simulink model "DoubleJoints_Algorithm"  (R2018b)
settings: Solver=FixedStepDiscrete  StartTime=0.0  StopTime=Inf  FixedStep=0.001  RelTol=1e-3  EnableMultiTasking=on
undefined symbols (not defined in the file): J2, J7, Motor_Current, Motor_Position, Motor_Velocity, Send_GUIdata
libraries: c280xlib x20, simulink x9, dspsrcs4 x2, idelinklib_common x1
(part 1 of 3)
settings Model: ExtModeTrigDuration=8  Creator=jeason  LastModifiedBy=Jeason
settings SolverCC: AutoInsertRateTranBlk=on
settings OptimizationCC: DefaultUnderspecifiedDataType=single  EnhancedBackFolding=on  PassReuseOutputArgsAs=Individual arguments  MaxStackSize=512  OptimizeBlockOrder=speed  DifferentSizesBufferReuse=on  OptimizationCustomize=off
settings DebuggingCC: MultiTaskDSMMsg=none  ParameterTunabilityLossMsg=error
settings HardwareCC: ProdBitPerChar=16  ProdBitPerInt=16  ProdBitPerPointer=32  ProdBitPerSizeT=32  ProdBitPerPtrDiffT=32  ProdLargestAtomicInteger=Integer  ProdLargestAtomicFloat=None  ProdWordSize=16  ProdLongLongMode=on  ProdHWDeviceType=Texas Instruments->C2000
settings SFSimCC: MATLABDynamicMemAlloc=off
settings RTWCC: SystemTargetFile=ert.tlc  HardwareBoard=TI Delfino F2833x  TemplateMakefile=ert_default_tmf  GenerateReport=on  Toolchain=Texas Instruments Code Composer Studio (C2000)  IncludeHyperlinkInReport=on  LaunchReport=on  GenerateTraceInfo=on  GenerateTraceReport=on  GenerateTraceReportSl=on  GenerateTraceReportSf=on  GenerateTraceReportEml=on
settings CodeAppCC: ForceParamTrailComments=on  IgnoreCustomStorageClasses=off  OperatorAnnotations=on  SimulinkDataObjDesc=on  SFDataObjDesc=on  InsertBlockDesc=on
settings ERTTargetCC: CodeReplacementLibrary=TI C28x

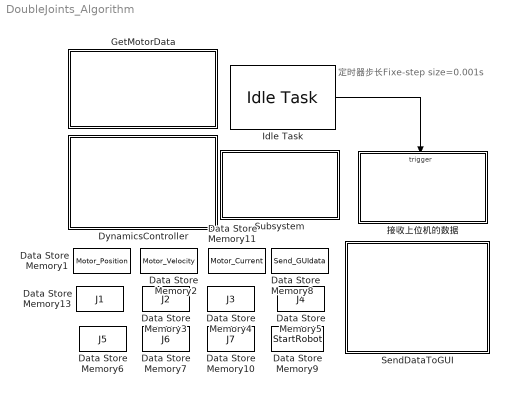
== system DoubleJoints_Algorithm ==
  note: 定时器步长Fixe-step size=0.001s
  Data Store Memory1 : DataStoreMemory  DataStoreName=Motor_Position  ReadBeforeWriteMsg=warning  WriteAfterWriteMsg=warning  WriteAfterReadMsg=warning  InitialValue=[0 0 0 0 0 0]  ShowAdditionalParam=off  OutDataTypeStr=int32
      settings: RTWStateStorageClass=ExportedGlobal
  Data Store Memory10 : DataStoreMemory  DataStoreName=J7  ReadBeforeWriteMsg=warning  WriteAfterWriteMsg=warning  WriteAfterReadMsg=warning  InitialValue=[0 0 0 0 0 0]  ShowAdditionalParam=off  OutDataTypeStr=double
      settings: RTWStateStorageClass=ExportedGlobal
  Data Store Memory11 : DataStoreMemory  DataStoreName=Motor_Current  ReadBeforeWriteMsg=warning  WriteAfterWriteMsg=warning  WriteAfterReadMsg=warning  InitialValue=[0 0 0 0 0 0]  ShowAdditionalParam=off  OutDataTypeStr=int32
      settings: RTWStateStorageClass=ExportedGlobal
  Data Store Memory13 : DataStoreMemory  DataStoreName=J1  ReadBeforeWriteMsg=warning  WriteAfterWriteMsg=warning  WriteAfterReadMsg=warning  InitialValue=[0 0 0 0 0 0]  ShowAdditionalParam=off  OutDataTypeStr=double
      settings: RTWStateStorageClass=ExportedGlobal
  Data Store Memory2 : DataStoreMemory  DataStoreName=Motor_Velocity  ReadBeforeWriteMsg=warning  WriteAfterWriteMsg=warning  WriteAfterReadMsg=warning  InitialValue=[0 0 0 0 0 0]  ShowAdditionalParam=off  OutDataTypeStr=int32
      settings: RTWStateStorageClass=ExportedGlobal
  Data Store Memory3 : DataStoreMemory  DataStoreName=J2  ReadBeforeWriteMsg=warning  WriteAfterWriteMsg=warning  WriteAfterReadMsg=warning  InitialValue=[0 0 0 0 0 0]  ShowAdditionalParam=off  OutDataTypeStr=double
      settings: RTWStateStorageClass=ExportedGlobal
  Data Store Memory4 : DataStoreMemory  DataStoreName=J3  ReadBeforeWriteMsg=warning  WriteAfterWriteMsg=warning  WriteAfterReadMsg=warning  InitialValue=[0 0 0 0 0 0]  ShowAdditionalParam=off  OutDataTypeStr=double
      settings: RTWStateStorageClass=ExportedGlobal
  Data Store Memory5 : DataStoreMemory  DataStoreName=J4  ReadBeforeWriteMsg=warning  WriteAfterWriteMsg=warning  WriteAfterReadMsg=warning  InitialValue=[0 0 0 0 0 0]  ShowAdditionalParam=off  OutDataTypeStr=double
      settings: RTWStateStorageClass=ExportedGlobal
  Data Store Memory6 : DataStoreMemory  DataStoreName=J5  ReadBeforeWriteMsg=warning  WriteAfterWriteMsg=warning  WriteAfterReadMsg=warning  InitialValue=[0 0 0 0 0 0]  ShowAdditionalParam=off  OutDataTypeStr=double
      settings: RTWStateStorageClass=ExportedGlobal
  Data Store Memory7 : DataStoreMemory  DataStoreName=J6  ReadBeforeWriteMsg=warning  WriteAfterWriteMsg=warning  WriteAfterReadMsg=warning  InitialValue=[0 0 0 0 0 0]  ShowAdditionalParam=off  OutDataTypeStr=double
      settings: RTWStateStorageClass=ExportedGlobal
  Data Store Memory8 : DataStoreMemory  DataStoreName=Send_GUIdata  ReadBeforeWriteMsg=warning  WriteAfterWriteMsg=warning  WriteAfterReadMsg=warning  InitialValue=zeros(1,18)  ShowAdditionalParam=off  OutDataTypeStr=double
      settings: RTWStateStorageClass=ExportedGlobal
  Data Store Memory9 : DataStoreMemory  DataStoreName=StartRobot  ReadBeforeWriteMsg=warning  WriteAfterWriteMsg=warning  WriteAfterReadMsg=warning  ShowAdditionalParam=off  OutDataTypeStr=uint16
      settings: RTWStateStorageClass=ExportedGlobal
  DynamicsController : Subsystem  Tag=Calculated_Data  Priority=2  TreatAsAtomicUnit=on
      settings: RTWSystemCode=Nonreusable function  RTWFcnNameOpts=Use subsystem name  RTWFileNameOpts=Use subsystem name
      mask Display:
      | color('red')
      | disp('六轴双关节\n自适应算法动力学计算')
  GetMotorData : Subsystem  Tag=Get_Data  Priority=0  TreatAsAtomicUnit=on
      settings: RTWSystemCode=Nonreusable function
  Idle Task : idelinklib_common/Idle Task  tasknumbers=[0]  taskpriorities=100016  taskpreempts=[1]  showinput=off  simPriority=0
  SendDataToGUI : Subsystem  Priority=2  TreatAsAtomicUnit=on
      settings: RTWSystemCode=Nonreusable function
  Subsystem : Subsystem
      mask Display: disp('System\nInitialization');
  接收上位机的数据 : Subsystem  TreatAsAtomicUnit=on
  wires:
  Idle Task/1 -> 接收上位机的数据/Trigger

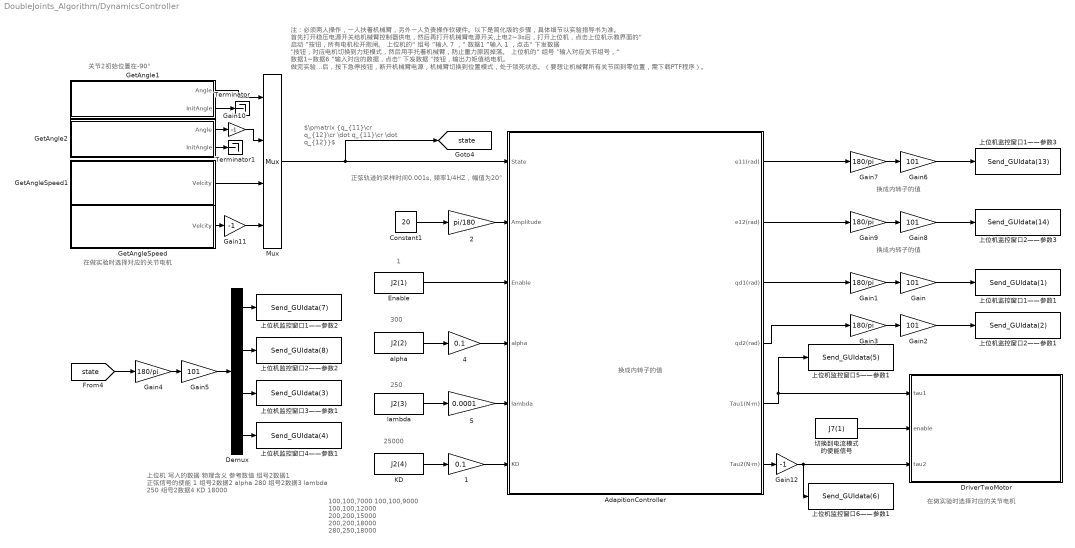
== system DoubleJoints_Algorithm/DynamicsController ==
  note: 100,100,7000
      | 100,100,9000
      | 100,100,12000
      | 200,200,15000
      | 200,200,18000
      | 280,250,18000
  note: 在做实验时选择对应的关节电机
  note: $\pmatrix {q_{11}\cr q_{12}\cr \dot q_{11}\cr \dot q_{12}}$
  note: 300
  note: 250
  note: 25000
  note: 1
  note: 在做实验时选择对应的关节电机
  note: 换成内转子的值
  note: 换成内转子的值
  note: 注：必须两人操作，一人扶着机械臂，另外一人负责操作软硬件。以下是简化版的步骤，具体细节以实验指导书为准。
      | 首先打开稳压电源开关给机械臂控制器供电，然后再打开机械臂电源开关,上电2~3s后，打开上位机，点击上位机示教界面的“ 启动 ”按钮，所有电机松开抱闸。
      | 上位机的“ 组号 ”输入 7 ，“ 数据1 ”输入 1 ，点击" 下发数据 "按钮，对应电机切换到力矩模式，然后用手托着机械臂，防止重力原因掉落。
      | 上位机的“ 组号 ”输入对应关节组号，“ 数据1~数据6 ”输入对应的数据，点击" 下发数据 "按钮，输出力矩值给电机。
      | 做完实验后，按下急停按钮，断开机械臂电源，机械臂切换到位置模式，处于锁死状态。（要想让机械臂所有关节回到零位置，需下载PTP程序）。
  note: 关节2初始位置在-90°
  note: 正弦轨迹的采样时间0.001s,
      | 频率1/4HZ，幅值为20°
  note: 上位机
      | 写入的数据
      | 物理含义
      | 参考数值
      |
      | 组号2数据1
      | 正弦信号的使能
      | 1
      |
      | 组号2数据2
      | alpha
      | 280
      |
      | 组号2数据3
      | lambda
      | 250
      |
      | 组号2数据4
      | KD
      | 18000
  note: 换成内转子的值
  1 : Gain  Gain=0.1  OutDataTypeStr=double
  2 : Gain  Gain=pi/180  OutDataTypeStr=double
  4 : Gain  Gain=0.1  OutDataTypeStr=double
  5 : Gain  Gain=0.0001  OutDataTypeStr=double
  AdapitionController : Subsystem  Priority=4  TreatAsAtomicUnit=on  RTWFcnName=AdapitionController  mask(双关节自适应算法控制器){Freq=1/4, SimpleTime=0.001}
      mask prompts: Freq "正弦信号的频率(HZ)"; SimpleTime "正弦信号的采样时间(s)"
      mask help:
      | 采样频率不能过快，否则机械臂摆动频率也会变快，至少为1/4.
      | 采样时间只能是定时器步长的整数倍，否则会报错，正弦信号的幅值最大为pi/3。
      settings: RTWSystemCode=Nonreusable function  RTWFcnNameOpts=User specified  RTWFileNameOpts=Use function name  FunctionInterfaceSpec=Allow arguments
      mask Display:
      | port_label('input', 1, 'State');
      | port_label('input', 2, '外转子正弦信号的幅值(rad)');
      | port_label('input', 3, '使能信号');
      | port_label('input', 4, 'alpha');
      | port_label('input', 5, 'lambda');
      | port_label('input', 6, 'KD');
      | 
      | port_label('output', 1, '关节2外转子跟踪误差(rad)');
      | port_label('output', 2, '关节3外转子跟踪误差(rad)');
      | port_label('output', 3, '关节2外转子理想正弦信号(rad)');
      | port_label('output', 4, '关节3外转子理想正弦信号(rad)');
      | port_label('output', 5, '关节2力矩Tau(N·m)');
      | port_label('output', 6, '关节3力矩Tau(N·m)');
  Constant1 : Constant  Value=20
  Demux : Demux
  DriverTwoMotor : Subsystem  TreatAsAtomicUnit=on  RTWFcnName=DriverTwoMotor  mask(驱动两个关节){SelectJoint1=2, SelectJoint2=3}
      mask prompts: SelectJoint1 "选择关节电机1"; SelectJoint2 "选择关节电机2"
      mask help:
      | 关节1~3为CANB,关节4~6为CANA,驱动的第一个电机的邮箱号为7，驱动的第二个电机的邮箱号为8。
      | 输入量的范围限定在-900~900。
      mask init:
      | vssBlk1_1 = [gcb, '/BottomDriver/Judgement/OneJoint/Joint1'];
      |     vssBlk1_2 = [gcb, '/BottomDriver/Judgement/OneJoint/Joint2'];
      |     vssBlk1_3 = [gcb, '/BottomDriver/Judgement/OneJoint/Joint3'];
      |     vssBlk1_4 = [gcb, '/BottomDriver/Judgement/OneJoint/Joint4'];
      |     vssBlk1_5 = [gcb, '/BottomDriver/Judgement/OneJoint/Joint5'];
      |     vssBlk1_6 = [gcb, '/BottomDriver/Judgement/OneJoint/Joint6'];
      |     vssBlk2_1 = [gcb, '/BottomDriver/Judgement/TwoJoint/Joint1'];
      |     vssBlk2_2 = [gcb, '/BottomDriver/Judgement/TwoJoint/Joint2'];
      |     vssBlk2_3 = [gcb, '/BottomDriver/Judgement/TwoJoint/Joint3'];
      |     vssBlk2_4 = [gcb, '/BottomDriver/Judgement/TwoJoint/Joint4'];
      |     vssBlk2_5 = [gcb, '/BottomDriver/Judgement/TwoJoint/Joint5'];
      |     vssBlk2_6 = [gcb, '/BottomDriver/Judgement/TwoJoint/Joint6'];
      |     choice1 = get_param(gcb,'SelectJoint1');
      |     choice2 = get_param(gcb,'SelectJoint2');
      |     if (strcmp(choice1,'1'))&&(strcmp(choice2,'1'))
      |         error('Error. Input can not be the same.');
      |     end
      |     if (strcmp(choice1,'2'))&&(strcmp(choice2,'2'))
      |         error('Error. Input can not be the same.');
      |     end
      |     if (strcmp(choice1,'3'))&&(strcmp(choice2,'3'))
      |         error('Error. Input can not be the same.');
      |     end
      |     if (strcmp(choice1,'4'))&&(strcmp(choice2,'4'))
      |         error('Error. Input can not be the same.');
      |     end
      |     if (strcmp(choice1,'5'))&&(strcmp(choice2,'5'))
      |         error('Error. Input can not be the same.');
      |     end
      |     if (strcmp(choice1,'6'))&&(strcmp(choice2,'6'))
      |         error('Error. Input can not be the same.');
      |     end
      |     clear choice1 vssBlk1_1 vssBlk1_2 vssBlk1_3 vssBlk1_4 vssBlk1_5 vssBlk1_6; 
      |     clear choice2 vssBlk2_1 vssBlk2_2 vssBlk2_3 vssBlk2_4 vssBlk2_5 vssBlk2_6;
      settings: RTWSystemCode=Nonreusable function  RTWFcnNameOpts=User specified  RTWFileNameOpts=Use function name  FunctionInterfaceSpec=Allow arguments  FunctionWithSeparateData=on
      mask TypeOptions SelectJoint1: 1 | 2 | 3 | 4 | 5 | 6
      mask Callback SelectJoint1:
      | vssBlk1_1 = [gcb, '/BottomDriver/Judgement/OneJoint/Joint1'];
      | vssBlk1_2 = [gcb, '/BottomDriver/Judgement/OneJoint/Joint2'];
      | vssBlk1_3 = [gcb, '/BottomDriver/Judgement/OneJoint/Joint3'];
      | vssBlk1_4 = [gcb, '/BottomDriver/Judgement/OneJoint/Joint4'];
      | vssBlk1_5 = [gcb, '/BottomDriver/Judgement/OneJoint/Joint5'];
      | vssBlk1_6 = [gcb, '/BottomDriver/Judgement/OneJoint/Joint6'];
      | choice1 = get_param(gcb,'SelectJoint1');
      | if strcmp(choice1,'1')
      |     set_param(vssBlk1_1, 'Commented','off');
      |     set_param(vssBlk1_2,'Commented','on');
      |     set_param(vssBlk1_3,'Commented','on');
      |     set_param(vssBlk1_4,'Commented','on');
      |     set_param(vssBlk1_5,'Commented','on');
      |     set_param(vssBlk1_6,'Commented','on');
      | elseif strcmp(choice1,'2')
      |     set_param(vssBlk1_2, 'Commented','off');
      |     set_param(vssBlk1_1,'Commented','on');
      |     set_param(vssBlk1_3,'Commented','on');
      |     set_param(vssBlk1_4,'Commented','on');
      |     set_param(vssBlk1_5,'Commented','on');
      |     set_param(vssBlk1_6,'Commented','on');
      | elseif strcmp(choice1,'3')
      |     set_param(vssBlk1_3, 'Commented','off');
      |     set_param(vssBlk1_1,'Commented','on');
      |     set_param(vssBlk1_2,'Commented','on');
      |     set_param(vssBlk1_4,'Commented','on');
      |     set_param(vssBlk1_5,'Commented','on');
      |     set_param(vssBlk1_6,'Commented','on');
      | elseif strcmp(choice1,'4')
      |     set_param(vssBlk1_4, 'Commented','off');
      |     set_param(vssBlk1_1,'Commented','on');
      |     set_param(vssBlk1_2,'Commented','on');
      |     set_param(vssBlk1_3,'Commented','on');
      |     set_param(vssBlk1_5,'Commented','on');
      |     set_param(vssBlk1_6,'Commented','on');
      | elseif strcmp(choice1,'5')
      |     set_param(vssBlk1_5, 'Commented','off');
      |     set_param(vssBlk1_1,'Commented','on');
      |     set_param(vssBlk1_2,'Commented','on');
      |     set_param(vssBlk1_3,'Commented','on');
      |     set_param(vssBlk1_4,'Commented','on');
      |     set_param(vssBlk1_6,'Commented','on');
      | elseif strcmp(choice1,'6')
      |     set_param(vssBlk1_6, 'Commented','off');
      |     set_param(vssBlk1_1,'Commented','on');
      |     set_param(vssBlk1_2,'Commented','on');
      |     set_param(vssBlk1_3,'Commented','on');
      |     set_param(vssBlk1_4,'Commented','on');
      |     set_param(vssBlk1_5,'Commented','on');
      | end
      | clear choice1 vssBlk1_1 vssBlk1_2 vssBlk1_3 vssBlk1_4 vssBlk1_5 vssBlk1_6;
      mask TypeOptions SelectJoint2: 1 | 2 | 3 | 4 | 5 | 6
      mask Callback SelectJoint2:
      | vssBlk2_1 = [gcb, '/BottomDriver/Judgement/TwoJoint/Joint1'];
      | vssBlk2_2 = [gcb, '/BottomDriver/Judgement/TwoJoint/Joint2'];
      | vssBlk2_3 = [gcb, '/BottomDriver/Judgement/TwoJoint/Joint3'];
      | vssBlk2_4 = [gcb, '/BottomDriver/Judgement/TwoJoint/Joint4'];
      | vssBlk2_5 = [gcb, '/BottomDriver/Judgement/TwoJoint/Joint5'];
      | vssBlk2_6 = [gcb, '/BottomDriver/Judgement/TwoJoint/Joint6'];
      | choice2 = get_param(gcb,'SelectJoint2');
      |  if strcmp(choice2,'1')
      |     set_param(vssBlk2_1, 'Commented','off');
      |     set_param(vssBlk2_2,'Commented','on');
      |     set_param(vssBlk2_3,'Commented','on');
      |     set_param(vssBlk2_4,'Commented','on');
      |     set_param(vssBlk2_5,'Commented','on');
      |     set_param(vssBlk2_6,'Commented','on');
      | elseif strcmp(choice2,'2')
      |     set_param(vssBlk2_2, 'Commented','off');
      |     set_param(vssBlk2_1,'Commented','on');
      |     set_param(vssBlk2_3,'Commented','on');
      |     set_param(vssBlk2_4,'Commented','on');
      |     set_param(vssBlk2_5,'Commented','on');
      |     set_param(vssBlk2_6,'Commented','on');
      | elseif strcmp(choice2,'3')
      |     set_param(vssBlk2_3, 'Commented','off');
      |     set_param(vssBlk2_1,'Commented','on');
      |     set_param(vssBlk2_2,'Commented','on');
      |     set_param(vssBlk2_4,'Commented','on');
      |     set_param(vssBlk2_5,'Commented','on');
      |     set_param(vssBlk2_6,'Commented','on');
      | elseif strcmp(choice2,'4')
      |     set_param(vssBlk2_4, 'Commented','off');
      |     set_param(vssBlk2_1,'Commented','on');
      |     set_param(vssBlk2_2,'Commented','on');
      |     set_param(vssBlk2_3,'Commented','on');
      |     set_param(vssBlk2_5,'Commented','on');
      |     set_param(vssBlk2_6,'Commented','on');
      | elseif strcmp(choice2,'5')
      |     set_param(vssBlk2_5, 'Commented','off');
      |     set_param(vssBlk2_1,'Commented','on');
      |     set_param(vssBlk2_2,'Commented','on');
      |     set_param(vssBlk2_3,'Commented','on');
      |     set_param(vssBlk2_4,'Commented','on');
      |     set_param(vssBlk2_6,'Commented','on');
      | elseif strcmp(choice2,'6')
      |     set_param(vssBlk2_6, 'Commented','off');
      |     set_param(vssBlk2_1,'Commented','on');
      |     set_param(vssBlk2_2,'Commented','on');
      |     set_param(vssBlk2_3,'Commented','on');
      |     set_param(vssBlk2_4,'Commented','on');
      |     set_param(vssBlk2_5,'Commented','on');
      | end
      | clear choice2 vssBlk2_1 vssBlk2_2 vssBlk2_3 vssBlk2_4 vssBlk2_5 vssBlk2_6;
      mask Display:
      | str1='双关节算法';str2='驱动关节'; str3='和';str4='电机';
      | choice1 = get_param(gcb,'SelectJoint1');
      | choice2 = get_param(gcb,'SelectJoint2');
      | str=[str1,'\n',str2,choice1,str3,choice2,str4];
      | disp(str);
      | port_label('input', 1, 'Tau1');
      | port_label('input', 2, 'Enable');
      | port_label('input', 3, 'Tau2');
  Enable : DataStoreRead  DataStoreName=J2  DataStoreElements=J2(1)
  Gain{,2,5..6,8} (5 alike) : Gain  Gain=101
  Gain{1,3..4,7,9} (5 alike) : Gain  Gain=180/pi
  Gain10 : Gain  Gain=-1
  Gain11 : Gain  Gain=-1
  Gain12 : Gain  Gain=-1
  GetAngle1 : Subsystem  TreatAsAtomicUnit=on  mask(获取电机外转子角度(rad)){JJoint=2, InitAngle=-90}
      mask prompts: JJoint "选择关节电机"; InitAngle "给定初始角度(deg)"
      mask help:
      | 给定初始角度：假设在数学建模时，设定连杆在水平位置为0°，而机械臂每个关节在出厂时都设定在竖直位置为0°，那么这里就需要给定一个偏置值90°/-90°，默认设为0。
      | 注：关节3因为结构原因实际获取到的角度的正负和标签贴的方向相反。
      | Angle(rad)=电机外转子的实际角度值-给定的初始角度值
      | InitAngle(rad)=给定的初始角度值
      mask TypeOptions JJoint: 1 | 2 | 3 | 4 | 5 | 6
      mask Display:
      | choice1 = get_param(gcb,'JJoint');
      | color('black');
      | switch choice1
      |     case '1'
      |         disp('获取关节1电机\n外转子角度(rad)');
      |     case '2'
      |         disp('获取关节2电机\n外转子角度(rad)');
      |     case '3'
      |         disp('获取关节3电机\n外转子角度(rad)');
      |     case '4'
      |         disp('获取关节4电机\n外转子角度(rad)');
      |     case '5'
      |         disp('获取关节5电机\n外转子角度(rad)');
      |     case '6'
      |         disp('获取关节6电机\n外转子角度(rad)');
      | end
      | color('black');
      | port_label('output', 1, 'Angle');
      | port_label('output', 2, 'InitAngle');
      | clear choice1;
  GetAngle2 : Subsystem  TreatAsAtomicUnit=on  mask(获取电机外转子角度(rad)){JJoint=3, InitAngle=0}
      mask prompts: JJoint "选择关节电机"; InitAngle "给定初始角度(deg)"
      mask help:
      | 给定初始角度：假设在数学建模时，设定连杆在水平位置为0°，而机械臂每个关节在出厂时都设定在竖直位置为0°，那么这里就需要给定一个偏置值90°/-90°，默认设为0。
      | 注：关节3因为结构原因实际获取到的角度的正负和标签贴的方向相反。
      | Angle(rad)=电机外转子的实际角度值-给定的初始角度值
      | InitAngle(rad)=给定的初始角度值
      mask TypeOptions JJoint: 1 | 2 | 3 | 4 | 5 | 6
      mask Display:
      | choice1 = get_param(gcb,'JJoint');
      | color('black');
      | switch choice1
      |     case '1'
      |         disp('获取关节1电机\n外转子角度(rad)');
      |     case '2'
      |         disp('获取关节2电机\n外转子角度(rad)');
      |     case '3'
      |         disp('获取关节3电机\n外转子角度(rad)');
      |     case '4'
      |         disp('获取关节4电机\n外转子角度(rad)');
      |     case '5'
      |         disp('获取关节5电机\n外转子角度(rad)');
      |     case '6'
      |         disp('获取关节6电机\n外转子角度(rad)');
      | end
      | color('black');
      | port_label('output', 1, 'Angle');
      | port_label('output', 2, 'InitAngle');
      | clear choice1;
  GetAngleSpeed : Subsystem  TreatAsAtomicUnit=on  mask{JJoint=3}
      mask prompts: JJoint "选择关节电机"
      mask help: 读取电机角速度(rad/s)
      mask TypeOptions JJoint: 1 | 2 | 3 | 4 | 5 | 6
      mask Display:
      | choice1 = get_param(gcb,'JJoint');
      | color('black');
      | switch choice1
      |     case '1'
      |         disp('获取关节1电机\n外转子角速度(rad/s)');
      |     case '2'
      |         disp('获取关节2电机\n外转子角速度(rad/s)');
      |     case '3'
      |         disp('获取关节3电机\n外转子角速度(rad/s)');
      |     case '4'
      |         disp('获取关节4电机\n外转子角速度(rad/s)');
      |     case '5'
      |         disp('获取关节5电机\n外转子角速度(rad/s)');
      |     case '6'
      |         disp('获取关节6电机\n外转子角速度(rad/s)');
      | end
      | color('black');
      | port_label('output', 1, 'Velocity');
      | clear choice1;
  GetAngleSpeed1 : Subsystem  TreatAsAtomicUnit=on  mask{JJoint=2}
      mask prompts: JJoint "选择关节电机"
      mask help: 读取电机角速度(rad/s)
      mask TypeOptions JJoint: 1 | 2 | 3 | 4 | 5 | 6
      mask Display:
      | choice1 = get_param(gcb,'JJoint');
      | color('black');
      | switch choice1
      |     case '1'
      |         disp('获取关节1电机\n外转子角速度(rad/s)');
      |     case '2'
      |         disp('获取关节2电机\n外转子角速度(rad/s)');
      |     case '3'
      |         disp('获取关节3电机\n外转子角速度(rad/s)');
      |     case '4'
      |         disp('获取关节4电机\n外转子角速度(rad/s)');
      |     case '5'
      |         disp('获取关节5电机\n外转子角速度(rad/s)');
      |     case '6'
      |         disp('获取关节6电机\n外转子角速度(rad/s)');
      | end
      | color('black');
      | port_label('output', 1, 'Velocity');
      | clear choice1;
  KD : DataStoreRead  DataStoreName=J2  DataStoreElements=J2(4)
  Mux : Mux
  Terminator : Terminator
  Terminator1 : Terminator
  alpha : DataStoreRead  DataStoreName=J2  DataStoreElements=J2(2)
  lambda : DataStoreRead  DataStoreName=J2  DataStoreElements=J2(3)
  上位机监控窗口1——参数1 : DataStoreWrite  DataStoreName=Send_GUIdata  DataStoreElements=Send_GUIdata(1)
  上位机监控窗口1——参数2 : DataStoreWrite  DataStoreName=Send_GUIdata  DataStoreElements=Send_GUIdata(7)
  上位机监控窗口1——参数3 : DataStoreWrite  DataStoreName=Send_GUIdata  DataStoreElements=Send_GUIdata(13)
  上位机监控窗口2——参数1 : DataStoreWrite  DataStoreName=Send_GUIdata  DataStoreElements=Send_GUIdata(2)
  上位机监控窗口2——参数2 : DataStoreWrite  DataStoreName=Send_GUIdata  DataStoreElements=Send_GUIdata(8)
  上位机监控窗口2——参数3 : DataStoreWrite  DataStoreName=Send_GUIdata  DataStoreElements=Send_GUIdata(14)
  上位机监控窗口3——参数1 : DataStoreWrite  DataStoreName=Send_GUIdata  DataStoreElements=Send_GUIdata(3)
  上位机监控窗口4——参数1 : DataStoreWrite  DataStoreName=Send_GUIdata  DataStoreElements=Send_GUIdata(4)
  上位机监控窗口5——参数1 : DataStoreWrite  DataStoreName=Send_GUIdata  DataStoreElements=Send_GUIdata(5)
  上位机监控窗口6——参数1 : DataStoreWrite  DataStoreName=Send_GUIdata  DataStoreElements=Send_GUIdata(6)
  切换到电流模式 的使能信号 : DataStoreRead  DataStoreName=J7  DataStoreElements=J7(1)
  tag scope: state=global
  wires:
  KD/1 -> 1/1
  Constant1/1 -> 2/1
  GetAngle1/1(Angle) -> Mux/1
  GetAngleSpeed1/1(Velcity) -> Mux/3
  GetAngleSpeed/1(Velcity) -> Gain11/1
  切换到电流模式 的使能信号/1 -> DriverTwoMotor/2(enable)
  Gain1/1 -> Gain/1
  Gain/1 -> 上位机监控窗口1——参数1/1
  Gain3/1 -> Gain2/1
  Gain2/1 -> 上位机监控窗口2——参数1/1
  Demux/1 -> 上位机监控窗口1——参数2/1
  Demux/2 -> 上位机监控窗口2——参数2/1
  [state] -> Gain4/1
  Gain4/1 -> Gain5/1
  Gain5/1 -> Demux/1
  Gain9/1 -> Gain8/1
  Gain7/1 -> Gain6/1
  Gain6/1 -> 上位机监控窗口1——参数3/1
  Gain8/1 -> 上位机监控窗口2——参数3/1
  Demux/4 -> 上位机监控窗口4——参数1/1
  Demux/3 -> 上位机监控窗口3——参数1/1
  AdapitionController/6(Tau2(N·m)) -> Gain12/1
  AdapitionController/5(Tau1(N·m)) -> DriverTwoMotor/1(tau1), 上位机监控窗口5——参数1/1
  Mux/1 -> AdapitionController/1(State), [state]
  2/1 -> AdapitionController/2(Amplitude)
  4/1 -> AdapitionController/4(alpha)
  5/1 -> AdapitionController/5(lambda)
  1/1 -> AdapitionController/6(KD)
  AdapitionController/1(e11(rad)) -> Gain7/1
  AdapitionController/2(e12(rad)) -> Gain9/1
  AdapitionController/3(qd1(rad)) -> Gain1/1
  AdapitionController/4(qd2(rad)) -> Gain3/1
  Gain10/1 -> Mux/2
  Gain11/1 -> Mux/4
  Gain12/1 -> DriverTwoMotor/3(tau2), 上位机监控窗口6——参数1/1
  lambda/1 -> 5/1
  alpha/1 -> 4/1
  Enable/1 -> AdapitionController/3(Enable)
  GetAngle2/1(Angle) -> Gain10/1
  GetAngle1/2(InitAngle) -> Terminator/1
  GetAngle2/2(InitAngle) -> Terminator1/1

== system DoubleJoints_Algorithm/GetMotorData ==
  note: 获取关节电流、 角速度、 角度信息
  CANA_284_24 : Subsystem  Priority=4  TreatAsAtomicUnit=on
      settings: RTWSystemCode=Nonreusable function
      mask Display:
      | color('WHITE')
      | disp('JOINT4\n数据读取')
  CANA_285_25 : Subsystem  Priority=5  TreatAsAtomicUnit=on
      settings: RTWSystemCode=Nonreusable function
      mask Display:
      | color('WHITE')
      | disp('JOINT5\n数据读取')
  CANA_286_26 : Subsystem  Priority=6  TreatAsAtomicUnit=on
      settings: RTWSystemCode=Nonreusable function
      mask Display:
      | color('WHITE')
      | disp('JOINT6\n数据读取')
  CANB_281_21 : Subsystem  Priority=1  TreatAsAtomicUnit=on
      settings: RTWSystemCode=Nonreusable function
      mask Display:
      | color('WHITE')
      | disp('JOINT1\n数据读取')
  CANB_282_22 : Subsystem  Priority=2  TreatAsAtomicUnit=on
      settings: RTWSystemCode=Nonreusable function
      mask Display:
      | color('white')
      | disp('JOINT2\n数据读取')
  CANB_283_23 : Subsystem  Priority=3  TreatAsAtomicUnit=on
      settings: RTWSystemCode=Nonreusable function
      mask Display:
      | color('white')
      | disp('JOINT3\n数据读取')

== system DoubleJoints_Algorithm/SendDataToGUI ==
  note: Upper limit=9
  note: 发送数据给上位机
  note: 定时器步长Fixe-step size=0.001s,
      | 每10ms发送一次数据给上位机
  " " : Subsystem
  Constant : Constant  Value=true  OutDataTypeStr=boolean
  Constant1 : Constant  Value=false  OutDataTypeStr=boolean
  Switch : Switch  Criteria=u2 > Threshold
  广播周期 : simulink/Sources/Counter Limited  uplimit=9  tsamp=-1
  wires:
  Switch/1 -> " "/Enable
  广播周期/1 -> Switch/2
  Constant1/1 -> Switch/1
  Constant/1 -> Switch/3

== system DoubleJoints_Algorithm/Subsystem ==
  Model Header : Subsystem  mask(Model Header){ShowInLibBrowser=0}
      mask prompts: ShowInLibBrowser "Simulink:masks:CustCodeMaskParam1_MP"
      settings: CopyFcn=cccopyfcn(gcb)  OpenFcn=ccopenfcn('Model Header')
      mask Help: eval('feval(''rtwprivate'',''rtwhelpview'',''rtw_model_header_block'')');
      mask Display: disp('Model\nHeader');
  Model Source : Subsystem  mask(Model Source){ShowInLibBrowser=0}
      mask prompts: ShowInLibBrowser "Simulink:masks:CustCodeMaskParam1_MP"
      settings: CopyFcn=cccopyfcn(gcb)  OpenFcn=ccopenfcn('Model Source')
      mask Help: eval('feval(''rtwprivate'',''rtwhelpview'',''rtw_model_source_block'')');
      mask Display: disp('Model\nSource');
  System Initialize : Subsystem  mask(System Initialize){ShowInLibBrowser=0}
      mask prompts: ShowInLibBrowser "Simulink:masks:CustCodeMaskParam1_MP"
      settings: CopyFcn=cccopyfcn(gcb)  OpenFcn=ccopenfcn('System Initialize Function')
      mask Help: eval('feval(''rtwprivate'',''rtwhelpview'',''rtw_sys_initialize_block'')');
      mask Display: disp('System\nInitialize');

== system DoubleJoints_Algorithm/接收上位机的数据 ==
  note: 接收上位机数据
  function : TriggerPort  TriggerType=function-call  VariantControl=Variant
  0x0080 : simulink/Logic and Bit Operations/Compare To Constant  relop===  const=hex2dec('0080')  OutDataTypeStr=boolean
  0x88 : simulink/Logic and Bit Operations/Compare To Constant  relop===  const=hex2dec('0088')  OutDataTypeStr=boolean
  Compare To Constant1 : simulink/Logic and Bit Operations/Compare To Constant  relop===  const=hex2dec('0001')  OutDataTypeStr=boolean
  Compare To Constant2 : simulink/Logic and Bit Operations/Compare To Constant  relop===  const=hex2dec('0001')  OutDataTypeStr=boolean
  Data Store Read : DataStoreRead  DataStoreName=PTX
  Data Store Write2 : DataStoreWrite  DataStoreName=StartRobot
  Data Type Conversion : DataTypeConversion  OutDataTypeStr=int16
  Data Type Conversion3 : DataTypeConversion  OutDataTypeStr=double
  Data Type Conversion4 : DataTypeConversion  OutDataTypeStr=uint16
  Demux1 : Demux  Outputs=9
  Logical Operator : Logic  Inputs=4  AllPortsSameDT=off  OutDataTypeStr=boolean
  Mux1 : Mux  Inputs=6
  Subsystem : Subsystem
  Terminator3 : Terminator
  消息使能 : DataStoreMemory  DataStoreName=PTX  ReadBeforeWriteMsg=warning  WriteAfterWriteMsg=warning  WriteAfterReadMsg=warning  InitialValue=true  ShowAdditionalParam=off  OutDataTypeStr=boolean
  获取用户命令 : Subsystem  Priority=1  TreatAsAtomicUnit=on
      settings: RTWSystemCode=Nonreusable function
  wires:
  Compare To Constant2/1 -> Logical Operator/4
  Compare To Constant1/1 -> Logical Operator/3
  Data Store Read/1 -> Logical Operator/2
  Logical Operator/1 -> Data Type Conversion4/1
  0x0080/1 -> Logical Operator/1
  Demux1/4 -> Mux1/2, Compare To Constant2/1
  Demux1/3 -> Mux1/1, Compare To Constant1/1
  Demux1/1 -> 0x0080/1, 0x88/1
  获取用户命令/1(消息) -> Demux1/1
  Demux1/5 -> Mux1/3
  Demux1/6 -> Mux1/4
  Demux1/9 -> Terminator3/1
  Demux1/7 -> Mux1/5
  Demux1/8 -> Mux1/6
  Mux1/1 -> Data Type Conversion/1
  Data Type Conversion/1 -> Data Type Conversion3/1
  Data Type Conversion4/1 -> Data Store Write2/1
  Demux1/2 -> Subsystem/1(组号)
  Data Type Conversion3/1 -> Subsystem/2(数据)
  0x88/1 -> Subsystem/Enable

== system DoubleJoints_Algorithm/DynamicsController/AdapitionController ==
  State : Inport
  Amplitude : Inport  Port=2
  Enable : Inport  Port=3
  alpha : Inport  Port=4
  lambda : Inport  Port=5
  KD : Inport  Port=6
  Controller : Subsystem  Priority=1  TreatAsAtomicUnit=on
      settings: RTWSystemCode=Nonreusable function  FunctionInterfaceSpec=Allow arguments
  "Error " : Subsystem  Priority=0  TreatAsAtomicUnit=on
      settings: RTWSystemCode=Nonreusable function  FunctionInterfaceSpec=Allow arguments
  Saturation : Saturate  UpperLimit=pi/3  LowerLimit=0
  e11(rad) : Outport
  e12(rad) : Outport  Port=2
  qd1(rad) : Outport  Port=3
  qd2(rad) : Outport  Port=4
  Tau1(N·m) : Outport  Port=5
  Tau2(N·m) : Outport  Port=6
  wires:
  "Error "/9(s1) -> Controller/6(s1)
  "Error "/7(ddqr1) -> Controller/4(ddqr_1)
  State/1 -> Controller/1(q), "Error "/1(state)
  Amplitude/1 -> Saturation/1
  "Error "/4(qd2) -> qd2(rad)/1
  "Error "/10(s2) -> Controller/7(s2)
  "Error "/8(ddqr2) -> Controller/5(ddqr_2)
  "Error "/5(dqr1) -> Controller/2(dqr_1)
  KD/1 -> Controller/9(KD)
  "Error "/6(dqr2) -> Controller/3(dqr_2)
  "Error "/3(qd1) -> qd1(rad)/1
  alpha/1 -> "Error "/4(alpha)
  lambda/1 -> Controller/8(lambda)
  Controller/2(tau2) -> Tau2(N·m)/1
  Controller/1(tau1) -> Tau1(N·m)/1
  Enable/1 -> "Error "/3(enable)
  "Error "/2(e12) -> e12(rad)/1
  "Error "/1(e11) -> e11(rad)/1
  Saturation/1 -> "Error "/2(gain)

== system DoubleJoints_Algorithm/DynamicsController/DriverTwoMotor ==
  tau1 : Inport
  enable : Inport  Port=2
  tau2 : Inport  Port=3
  BottomDriver : Subsystem  Priority=2
      settings: RTWSystemCode=Nonreusable function
  Constant1 : Constant  Value=SelectJoint1  OutDataTypeStr=uint8
  Constant2 : Constant  Value=SelectJoint2  OutDataTypeStr=uint8
  Data Store Memory2 : DataStoreMemory  DataStoreName=TWO_TXD  ReadBeforeWriteMsg=warning  WriteAfterWriteMsg=warning  WriteAfterReadMsg=warning  InitialValue=[0]  ShowAdditionalParam=off  OutDataTypeStr=uint8
      settings: RTWStateStorageClass=ExportedGlobal
  Data Store Read4 : DataStoreRead  DataStoreName=TWO_TXD
  限幅 : Saturate  UpperLimit=900  LowerLimit=-900
  限幅1 : Saturate  UpperLimit=900  LowerLimit=-900
  驱动器指令 : Subsystem  Priority=1  TreatAsAtomicUnit=on
      settings: RTWSystemCode=Nonreusable function
  wires:
  tau2/1 -> 限幅/1
  限幅/1 -> 驱动器指令/2(Current2)
  Constant1/1 -> BottomDriver/1(SelectJoint1)
  Data Store Read4/1 -> BottomDriver/Enable
  tau1/1 -> 限幅1/1
  限幅1/1 -> 驱动器指令/1(Current1)
  Constant2/1 -> BottomDriver/2(SelectJoint2)
  enable/1 -> 驱动器指令/3(enable)
  驱动器指令/1(MSG1) -> BottomDriver/3(MSG1)
  驱动器指令/2(MSG2) -> BottomDriver/4(MSG2)

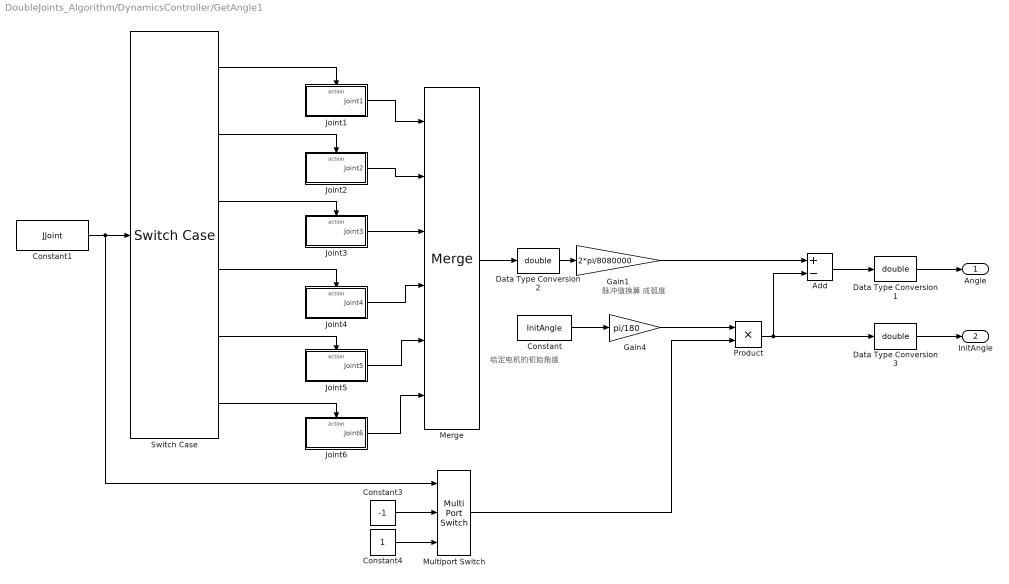
== system DoubleJoints_Algorithm/DynamicsController/GetAngle1 ==
  note: 脉冲值换算
      | 成弧度
  note: 给定电机的初始角度
  Add : Sum  Inputs=+-
  Constant : Constant  Value=InitAngle
  Constant1 : Constant  Value=JJoint  OutDataTypeStr=uint8
  Constant3 : Constant  Value=-1
  Constant4 : Constant
  Data Type Conversion1 : DataTypeConversion  OutDataTypeStr=double
  Data Type Conversion2 : DataTypeConversion  OutDataTypeStr=double
  Data Type Conversion3 : DataTypeConversion  OutDataTypeStr=double
  Gain1 : Gain  Gain=2*pi/8080000
  Gain4 : Gain  Gain=pi/180
  Joint1 : Subsystem  TreatAsAtomicUnit=on
  Joint2 : Subsystem  TreatAsAtomicUnit=on
  Joint3 : Subsystem  TreatAsAtomicUnit=on
  Joint4 : Subsystem  TreatAsAtomicUnit=on
  Joint5 : Subsystem  TreatAsAtomicUnit=on
  Joint6 : Subsystem  TreatAsAtomicUnit=on
  Merge : Merge  Inputs=6  InitialOutput=0
  Multiport Switch : MultiPortSwitch  DataPortOrder=Specify indices  Inputs=2  DataPortIndices={3,[1,2,4,5,6]}
  Product : Product
  Switch Case : SwitchCase  CaseConditions={1 2 3 4 5 6}  ShowDefaultCase=off
  Angle : Outport
  InitAngle : Outport  Port=2
  wires:
  Data Type Conversion2/1 -> Gain1/1
  Data Type Conversion1/1 -> Angle/1
  Joint6/1(Joint6) -> Merge/6
  Joint5/1(Joint5) -> Merge/5
  Joint4/1(Joint4) -> Merge/4
  Joint3/1(Joint3) -> Merge/3
  Joint2/1(Joint2) -> Merge/2
  Joint1/1(Joint1) -> Merge/1
  Switch Case/6 -> Joint6/Action
  Switch Case/5 -> Joint5/Action
  Switch Case/4 -> Joint4/Action
  Switch Case/3 -> Joint3/Action
  Switch Case/2 -> Joint2/Action
  Switch Case/1 -> Joint1/Action
  Constant/1 -> Gain4/1
  Add/1 -> Data Type Conversion1/1
  Gain1/1 -> Add/1
  Gain4/1 -> Product/1
  Merge/1 -> Data Type Conversion2/1
  Multiport Switch/1 -> Product/2
  Constant4/1 -> Multiport Switch/3
  Constant3/1 -> Multiport Switch/2
  Constant1/1 -> Multiport Switch/1, Switch Case/1
  Product/1 -> Data Type Conversion3/1, Add/2
  Data Type Conversion3/1 -> InitAngle/1

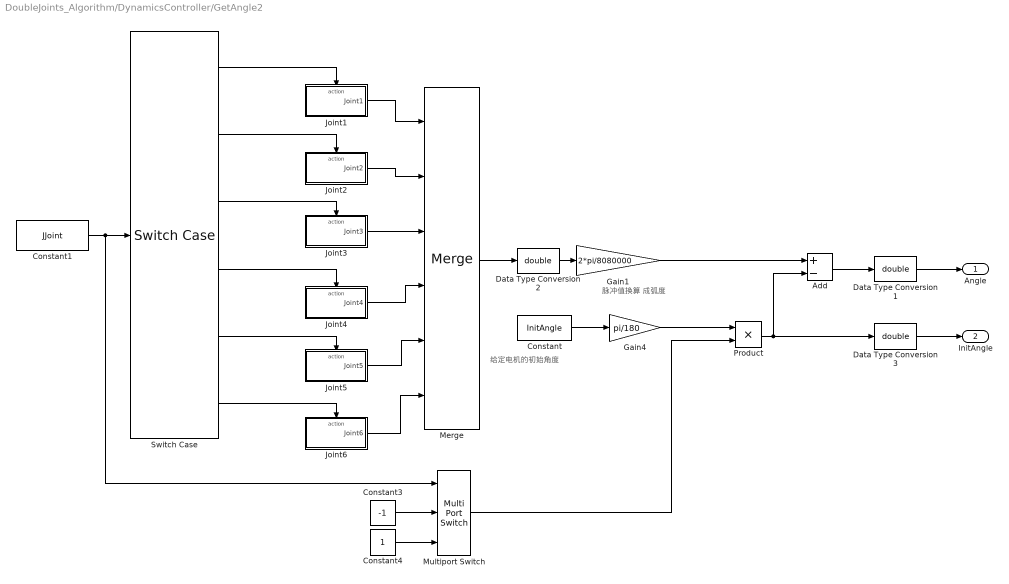
== system DoubleJoints_Algorithm/DynamicsController/GetAngle2 ==
  note: 给定电机的初始角度
  note: 脉冲值换算
      | 成弧度
  Add : Sum  Inputs=+-
  Constant : Constant  Value=InitAngle
  Constant1 : Constant  Value=JJoint  OutDataTypeStr=uint8
  Constant3 : Constant  Value=-1
  Constant4 : Constant
  Data Type Conversion1 : DataTypeConversion  OutDataTypeStr=double
  Data Type Conversion2 : DataTypeConversion  OutDataTypeStr=double
  Data Type Conversion3 : DataTypeConversion  OutDataTypeStr=double
  Gain1 : Gain  Gain=2*pi/8080000
  Gain4 : Gain  Gain=pi/180
  Joint1 : Subsystem  TreatAsAtomicUnit=on
  Joint2 : Subsystem  TreatAsAtomicUnit=on
  Joint3 : Subsystem  TreatAsAtomicUnit=on
  Joint4 : Subsystem  TreatAsAtomicUnit=on
  Joint5 : Subsystem  TreatAsAtomicUnit=on
  Joint6 : Subsystem  TreatAsAtomicUnit=on
  Merge : Merge  Inputs=6  InitialOutput=0
  Multiport Switch : MultiPortSwitch  DataPortOrder=Specify indices  Inputs=2  DataPortIndices={3,[1,2,4,5,6]}
  Product : Product
  Switch Case : SwitchCase  CaseConditions={1 2 3 4 5 6}  ShowDefaultCase=off
  Angle : Outport
  InitAngle : Outport  Port=2
  wires:
  Data Type Conversion3/1 -> InitAngle/1
  Product/1 -> Add/2, Data Type Conversion3/1
  Constant1/1 -> Switch Case/1, Multiport Switch/1
  Constant3/1 -> Multiport Switch/2
  Constant4/1 -> Multiport Switch/3
  Multiport Switch/1 -> Product/2
  Merge/1 -> Data Type Conversion2/1
  Gain4/1 -> Product/1
  Gain1/1 -> Add/1
  Add/1 -> Data Type Conversion1/1
  Constant/1 -> Gain4/1
  Switch Case/1 -> Joint1/Action
  Switch Case/2 -> Joint2/Action
  Switch Case/3 -> Joint3/Action
  Switch Case/4 -> Joint4/Action
  Switch Case/5 -> Joint5/Action
  Switch Case/6 -> Joint6/Action
  Joint1/1(Joint1) -> Merge/1
  Joint2/1(Joint2) -> Merge/2
  Joint3/1(Joint3) -> Merge/3
  Joint4/1(Joint4) -> Merge/4
  Joint5/1(Joint5) -> Merge/5
  Joint6/1(Joint6) -> Merge/6
  Data Type Conversion1/1 -> Angle/1
  Data Type Conversion2/1 -> Gain1/1

== system DoubleJoints_Algorithm/DynamicsController/GetAngleSpeed ==
  note: 换算成角速度2π/1min
  Constant1 : Constant  Value=JJoint
  Data Type Conversion3 : DataTypeConversion  OutDataTypeStr=double
  Gain3 : Gain  Gain=2*pi/60
  Gain9 : Gain  Gain=1/101
  Joint1 : Subsystem  TreatAsAtomicUnit=on
  Joint2 : Subsystem  TreatAsAtomicUnit=on
  Joint3 : Subsystem  TreatAsAtomicUnit=on
  Joint4 : Subsystem  TreatAsAtomicUnit=on
  Joint5 : Subsystem  TreatAsAtomicUnit=on
  Joint6 : Subsystem  TreatAsAtomicUnit=on
  Merge1 : Merge  Inputs=6  InitialOutput=0
  Switch Case : SwitchCase  CaseConditions={1 2 3 4 5 6}  ShowDefaultCase=off
  Velcity : Outport
  wires:
  Constant1/1 -> Switch Case/1
  Switch Case/1 -> Joint1/Action
  Switch Case/2 -> Joint2/Action
  Switch Case/3 -> Joint3/Action
  Switch Case/4 -> Joint4/Action
  Switch Case/5 -> Joint5/Action
  Switch Case/6 -> Joint6/Action
  Data Type Conversion3/1 -> Gain3/1
  Joint6/1(Joint6_Velocity) -> Merge1/6
  Joint5/1(Joint5_Velocity) -> Merge1/5
  Joint4/1(Joint4_Velocity) -> Merge1/4
  Joint3/1(Joint3_Velocity) -> Merge1/3
  Joint2/1(Joint2_Velocity) -> Merge1/2
  Joint1/1(Joint1_Velocity) -> Merge1/1
  Gain3/1 -> Gain9/1
  Gain9/1 -> Velcity/1
  Merge1/1 -> Data Type Conversion3/1

== system DoubleJoints_Algorithm/DynamicsController/GetAngleSpeed1 ==
  note: 换算成角速度2π/1min
  Constant1 : Constant  Value=JJoint
  Data Type Conversion3 : DataTypeConversion  OutDataTypeStr=double
  Gain3 : Gain  Gain=2*pi/60
  Gain9 : Gain  Gain=1/101
  Joint1 : Subsystem  TreatAsAtomicUnit=on
  Joint2 : Subsystem  TreatAsAtomicUnit=on
  Joint3 : Subsystem  TreatAsAtomicUnit=on
  Joint4 : Subsystem  TreatAsAtomicUnit=on
  Joint5 : Subsystem  TreatAsAtomicUnit=on
  Joint6 : Subsystem  TreatAsAtomicUnit=on
  Merge1 : Merge  Inputs=6  InitialOutput=0
  Switch Case : SwitchCase  CaseConditions={1 2 3 4 5 6}  ShowDefaultCase=off
  Velcity : Outport
  wires:
  Merge1/1 -> Data Type Conversion3/1
  Gain9/1 -> Velcity/1
  Gain3/1 -> Gain9/1
  Joint1/1(Joint1_Velocity) -> Merge1/1
  Joint2/1(Joint2_Velocity) -> Merge1/2
  Joint3/1(Joint3_Velocity) -> Merge1/3
  Joint4/1(Joint4_Velocity) -> Merge1/4
  Joint5/1(Joint5_Velocity) -> Merge1/5
  Joint6/1(Joint6_Velocity) -> Merge1/6
  Data Type Conversion3/1 -> Gain3/1
  Switch Case/6 -> Joint6/Action
  Switch Case/5 -> Joint5/Action
  Switch Case/4 -> Joint4/Action
  Switch Case/3 -> Joint3/Action
  Switch Case/2 -> Joint2/Action
  Switch Case/1 -> Joint1/Action
  Constant1/1 -> Switch Case/1

== system DoubleJoints_Algorithm/GetMotorData/CANA_284_24 ==
  note: 控制器接收ID:0x280+“ID”
  Subsystem1 : Subsystem
  eCAN Receive1 : c280xlib/eCAN Receive  chipFamily=C280x  useModule=eCAN_A  mailboxNo=24  messageID=hex2dec('284')  messageType=Standard (11-bit identifier)  sampleTime=-1  dataType=uint8  initValue=0  outputMessageLength=off  outputMessageTimeStamp=off  postInterrupt=off  interruptLine=0
      settings: SourceProductName=Embedded Coder Support Package for Texas Instruments C2000 Processors  SourceProductBaseCode=TIC2000
  wires:
  eCAN Receive1/2 -> Subsystem1/1(In1)
  eCAN Receive1/1 -> Subsystem1/Trigger

== system DoubleJoints_Algorithm/GetMotorData/CANA_285_25 ==
  note: 控制器接收ID:0x280+“ID”
  Subsystem : Subsystem
  eCAN Receive : c280xlib/eCAN Receive  chipFamily=C280x  useModule=eCAN_A  mailboxNo=25  messageID=hex2dec('285')  messageType=Standard (11-bit identifier)  sampleTime=-1  dataType=uint8  initValue=0  outputMessageLength=off  outputMessageTimeStamp=off  postInterrupt=off  interruptLine=0
      settings: SourceProductName=Embedded Coder Support Package for Texas Instruments C2000 Processors  SourceProductBaseCode=TIC2000
  wires:
  eCAN Receive/2 -> Subsystem/1(In1)
  eCAN Receive/1 -> Subsystem/Trigger

== system DoubleJoints_Algorithm/GetMotorData/CANA_286_26 ==
  note: 控制器接收ID:0x280+“ID”
  Subsystem : Subsystem
  eCAN Receive : c280xlib/eCAN Receive  chipFamily=C280x  useModule=eCAN_A  mailboxNo=26  messageID=hex2dec('286')  messageType=Standard (11-bit identifier)  sampleTime=-1  dataType=uint8  initValue=0  outputMessageLength=off  outputMessageTimeStamp=off  postInterrupt=off  interruptLine=0
      settings: SourceProductName=Embedded Coder Support Package for Texas Instruments C2000 Processors  SourceProductBaseCode=TIC2000
  wires:
  eCAN Receive/2 -> Subsystem/1(In1)
  eCAN Receive/1 -> Subsystem/Trigger

== system DoubleJoints_Algorithm/GetMotorData/CANB_281_21 ==
  note: 控制器接收ID:0x280+“ID”
  Subsystem : Subsystem
  eCAN Receive : c280xlib/eCAN Receive  chipFamily=C280x  useModule=eCAN_B  mailboxNo=21  messageID=hex2dec('281')  messageType=Standard (11-bit identifier)  sampleTime=-1  dataType=uint8  initValue=0  outputMessageLength=off  outputMessageTimeStamp=off  postInterrupt=off  interruptLine=0
      settings: SourceProductName=Embedded Coder Support Package for Texas Instruments C2000 Processors  SourceProductBaseCode=TIC2000
  wires:
  eCAN Receive/2 -> Subsystem/1(In1)
  eCAN Receive/1 -> Subsystem/Trigger

== system DoubleJoints_Algorithm/GetMotorData/CANB_282_22 ==
  note: 控制器接收ID:0x280+“ID”
  Subsystem : Subsystem
  eCAN Receive : c280xlib/eCAN Receive  chipFamily=C280x  useModule=eCAN_B  mailboxNo=22  messageID=hex2dec('282')  messageType=Standard (11-bit identifier)  sampleTime=-1  dataType=uint8  initValue=0  outputMessageLength=off  outputMessageTimeStamp=off  postInterrupt=off  interruptLine=0
      settings: SourceProductName=Embedded Coder Support Package for Texas Instruments C2000 Processors  SourceProductBaseCode=TIC2000
  wires:
  eCAN Receive/2 -> Subsystem/1(In1)
  eCAN Receive/1 -> Subsystem/Trigger

== system DoubleJoints_Algorithm/GetMotorData/CANB_283_23 ==
  note: 控制器接收ID:0x280+“ID”
  Subsystem : Subsystem
  eCAN Receive : c280xlib/eCAN Receive  chipFamily=C280x  useModule=eCAN_B  mailboxNo=23  messageID=hex2dec('283')  messageType=Standard (11-bit identifier)  sampleTime=-1  dataType=uint8  initValue=0  outputMessageLength=off  outputMessageTimeStamp=off  postInterrupt=off  interruptLine=0
      settings: SourceProductName=Embedded Coder Support Package for Texas Instruments C2000 Processors  SourceProductBaseCode=TIC2000
  wires:
  eCAN Receive/2 -> Subsystem/1(In1)
  eCAN Receive/1 -> Subsystem/Trigger

== system DoubleJoints_Algorithm/SendDataToGUI/  ==
  Enable : EnablePort
  Constant1 : Constant  Value=hex2dec('5a')  OutDataTypeStr=uint16
  Data Store Read4 : DataStoreRead  DataStoreName=Send_GUIdata
  Data Type Conversion12 : DataTypeConversion  OutDataTypeStr=uint16
  Demux : Demux  Outputs=18
  Mux : Mux  Inputs=20
  SCI Transmit : c280xlib/SCI Transmit  sciModule=A  dataHead=''  dataTail=''  postInterrupt=off  numFifo=1
      settings: SourceProductName=Embedded Coder Support Package for Texas Instruments C2000 Processors
  校验码填充 : Sum  Inputs=+++++++++++++++++++  AccumDataTypeStr=uint16
  wires:
  Demux/1 -> Mux/2, 校验码填充/2
  Mux/1 -> SCI Transmit/1
  Demux/3 -> 校验码填充/4, Mux/4
  Demux/14 -> 校验码填充/15, Mux/15
  Demux/9 -> 校验码填充/10, Mux/10
  Demux/5 -> Mux/6, 校验码填充/6
  Demux/2 -> 校验码填充/3, Mux/3
  Data Store Read4/1 -> Data Type Conversion12/1
  Demux/13 -> 校验码填充/14, Mux/14
  Demux/6 -> Mux/7, 校验码填充/7
  Demux/8 -> 校验码填充/9, Mux/9
  Demux/10 -> 校验码填充/11, Mux/11
  Demux/4 -> 校验码填充/5, Mux/5
  Demux/7 -> 校验码填充/8, Mux/8
  Demux/15 -> 校验码填充/16, Mux/16
  Demux/11 -> 校验码填充/12, Mux/12
  Demux/18 -> 校验码填充/19, Mux/19
  Demux/16 -> 校验码填充/17, Mux/17
  Constant1/1 -> 校验码填充/1, Mux/1
  Demux/17 -> 校验码填充/18, Mux/18
  校验码填充/1 -> Mux/20
  Demux/12 -> 校验码填充/13, Mux/13
  Data Type Conversion12/1 -> Demux/1

== system DoubleJoints_Algorithm/Subsystem/Model Header ==

== system DoubleJoints_Algorithm/Subsystem/Model Source ==

== system DoubleJoints_Algorithm/Subsystem/System Initialize ==

== system DoubleJoints_Algorithm/接收上位机的数据/Subsystem ==
  组号 : Inport
  数据 : Inport  Port=2
  Enable : EnablePort
  Joint1 : Subsystem  TreatAsAtomicUnit=on
  Joint2 : Subsystem  TreatAsAtomicUnit=on
  Joint3 : Subsystem  TreatAsAtomicUnit=on
  Joint4 : Subsystem  TreatAsAtomicUnit=on
  Joint5 : Subsystem  TreatAsAtomicUnit=on
  Joint6 : Subsystem  TreatAsAtomicUnit=on
  Joint7 : Subsystem  TreatAsAtomicUnit=on
  Switch Case : SwitchCase  CaseConditions={1 2 3 4 5 6 7}  ShowDefaultCase=off
  wires:
  数据/1 -> Joint7/1(Joint7), Joint5/1(Joint5), Joint4/1(Joint4), Joint3/1(Joint3), Joint2/1(Joint2), Joint1/1(Joint1), Joint6/1(Joint6)
  Switch Case/5 -> Joint5/Action
  Switch Case/6 -> Joint6/Action
  Switch Case/2 -> Joint2/Action
  Switch Case/1 -> Joint1/Action
  Switch Case/3 -> Joint3/Action
  Switch Case/4 -> Joint4/Action
  组号/1 -> Switch Case/1
  Switch Case/7 -> Joint7/Action

== system DoubleJoints_Algorithm/接收上位机的数据/获取用户命令 ==
  " " : c280xlib/SCI Receive  sciModule=A  dataHead=''  dataTail=''  dataType=uint16  dataDim=9  initValue=0  errOption=Output the last received value  errValue=0  sampleTime=-1  outputStatus=on  postInterrupt=off  numFifo=1
      settings: SourceProductName=Embedded Coder Support Package for Texas Instruments C2000 Processors  SourceProductBaseCode=TIC2000
  Constant : Constant  Value=false  OutDataTypeStr=boolean
  Constant1 : Constant  Value=true  OutDataTypeStr=boolean
  Data Store Write1 : DataStoreWrite  DataStoreName=PTX
  Logical Operator : Logic  AllPortsSameDT=off  OutDataTypeStr=boolean
  Switch : Switch  Criteria=u2 > Threshold
  消息校验 : Subsystem
  消息 : Outport
  wires:
  消息校验/2(使能) -> Logical Operator/1
  Switch/1 -> Logical Operator/2
  Constant1/1 -> Switch/3
  " "/2 -> Switch/2
  消息校验/1(消息) -> 消息/1
  " "/1 -> 消息校验/1(数据)
  Logical Operator/1 -> Data Store Write1/1
  Constant/1 -> Switch/1

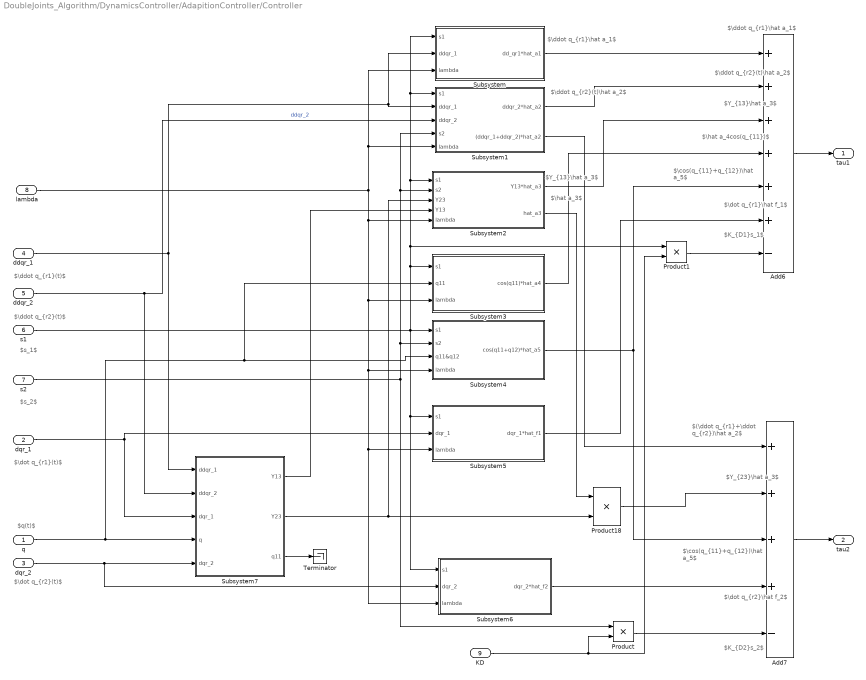
== system DoubleJoints_Algorithm/DynamicsController/AdapitionController/Controller ==
  note: $\ddot q_{r1}(t)$
  note: $\ddot q_{r2}(t)$
  note: $s_1$
  note: $\dot q_{r1}(t)$
  note: $\dot q_{r2}(t)$
  note: $q(t)$
  note: $\ddot q_{r1}\hat a_1$
  note: $s_2$
  note: $(\ddot q_{r1}+\ddot q_{r2})\hat a_2$
  note: $\hat a_3$
  note: $Y_{13}\hat a_3$
  note: $\ddot q_{r2}(t)\hat a_2$
  note: $\hat a_4cos(q_{11})$
  note: $\cos(q_{11}+q_{12})\hat a_5$
  note: $\dot q_{r1}\hat f_1$
  note: $K_{D1}s_1$
  note: $Y_{13}\hat a_3$
  note: $\ddot q_{r2}(t)\hat a_2$
  note: $\ddot q_{r1}\hat a_1$
  note: $Y_{23}\hat a_3$
  note: $\cos(q_{11}+q_{12})\hat a_5$
  note: $\dot q_{r2}\hat f_2$
  note: $K_{D2}s_2$
  q : Inport
  dqr_1 : Inport  Port=2
  dqr_2 : Inport  Port=3
  ddqr_1 : Inport  Port=4
  ddqr_2 : Inport  Port=5
  s1 : Inport  Port=6
  s2 : Inport  Port=7
  lambda : Inport  Port=8
  KD : Inport  Port=9
  Add6 : Sum  Inputs=++++++-
  Add7 : Sum  Inputs=++++-
  Product : Product
  Product1 : Product
  Product18 : Product
  Subsystem : Subsystem  TreatAsAtomicUnit=on
      settings: RTWSystemCode=Nonreusable function  FunctionInterfaceSpec=Allow arguments  FunctionWithSeparateData=on
  Subsystem1 : Subsystem  TreatAsAtomicUnit=on
      settings: RTWSystemCode=Nonreusable function  FunctionInterfaceSpec=Allow arguments  FunctionWithSeparateData=on
  Subsystem2 : Subsystem  TreatAsAtomicUnit=on
      settings: RTWSystemCode=Nonreusable function  FunctionInterfaceSpec=Allow arguments  FunctionWithSeparateData=on
  Subsystem3 : Subsystem  TreatAsAtomicUnit=on
      settings: RTWSystemCode=Nonreusable function  FunctionInterfaceSpec=Allow arguments  FunctionWithSeparateData=on
  Subsystem4 : Subsystem  TreatAsAtomicUnit=on
      settings: RTWSystemCode=Nonreusable function  FunctionInterfaceSpec=Allow arguments  FunctionWithSeparateData=on
  Subsystem5 : Subsystem  TreatAsAtomicUnit=on
      settings: RTWSystemCode=Nonreusable function  FunctionInterfaceSpec=Allow arguments  FunctionWithSeparateData=on
  Subsystem6 : Subsystem  TreatAsAtomicUnit=on
      settings: RTWSystemCode=Nonreusable function  FunctionInterfaceSpec=Allow arguments  FunctionWithSeparateData=on
  Subsystem7 : Subsystem  TreatAsAtomicUnit=on
      settings: RTWSystemCode=Nonreusable function  FunctionInterfaceSpec=Allow arguments  FunctionWithSeparateData=on
  Terminator : Terminator
  tau1 : Outport
  tau2 : Outport  Port=2
  wires:
  Product18/1 -> Add7/2
  dqr_2/1 -> Subsystem6/2(dqr_2), Subsystem7/5(dqr_2)
  q/1 -> Subsystem7/4(q), Subsystem3/2(q11), Subsystem4/3(q11&q12)
  ddqr_1/1 -> Subsystem7/1(ddqr_1), Subsystem/2(ddqr_1), Subsystem1/2(ddqr_1)
  ddqr_2/1 -> Subsystem1/3(ddqr_2), Subsystem7/2(ddqr_2)  "ddqr_2"
  dqr_1/1 -> Subsystem7/3(dqr_1), Subsystem5/2(dqr_1)
  Add6/1 -> tau1/1
  Add7/1 -> tau2/1
  Subsystem/1(dd_qr1*hat_a1) -> Add6/1
  s2/1 -> Product/1, Subsystem1/4(s2), Subsystem2/2(s2), Subsystem4/2(s2)
  Subsystem1/1(ddqr_2*hat_a2) -> Add6/2
  Subsystem1/2((ddqr_1+ddqr_2)*hat_a2) -> Add7/1
  Subsystem2/1(Y13*hat_a3) -> Add6/3
  Subsystem2/2(hat_a3) -> Product18/1
  Subsystem3/1(cos(q11)*hat_a4) -> Add6/4
  Subsystem4/1(cos(q11+q12)*hat_a5) -> Add6/5, Add7/3
  Subsystem5/1(dqr_1*hat_f1) -> Add6/6
  Subsystem6/1(dqr_2*hat_f2) -> Add7/4
  Product1/1 -> Add6/7
  s1/1 -> Subsystem/1(s1), Subsystem1/1(s1), Subsystem2/1(s1), Product1/1, Subsystem3/1(s1), Subsystem4/1(s1), Subsystem6/1(s1), Subsystem5/1(s1)
  Product/1 -> Add7/5
  Subsystem7/2("Y23 ") -> Subsystem2/3(Y23), Product18/2
  Subsystem7/1(Y13) -> Subsystem2/4(Y13)
  Subsystem7/3(q11) -> Terminator/1
  lambda/1 -> Subsystem6/3(lambda), Subsystem5/3(lambda), Subsystem4/4(lambda), Subsystem3/3(lambda), Subsystem2/5(lambda), Subsystem/3(lambda), Subsystem1/5(lambda)
  KD/1 -> Product1/2, Product/2
